simulink model "Levitador_aire_parametrizado"  (R2024b)
settings: Solver=VariableStepAuto  StartTime=0.0  StopTime=30  MaxStep=0.1  RelTol=1e-3
undefined symbols (not defined in the file): alfa, g, kd, kf, ki, kp, m, tao1, xi
libraries: slpidlib x1
settings Model: PacingRate=10  Creator=santiagolopez  LastModifiedBy=santiagolopez
settings DataIOCC: ReturnWorkspaceOutputs=off

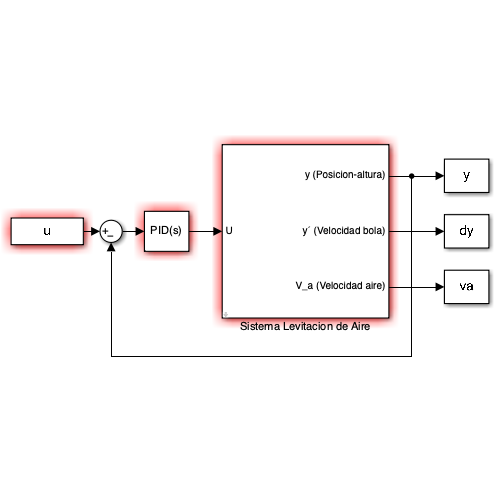
[thumbnail: Simulink's stored preview of the top-level diagram]
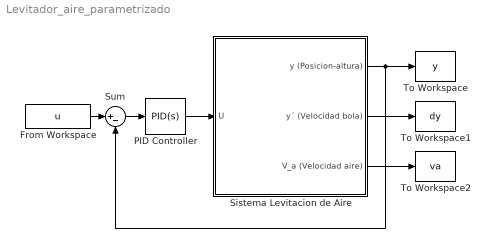
== system Levitador_aire_parametrizado ==
  From Workspace : FromWorkspace  VariableName=u
  PID Controller : slpidlib/PID Controller  Controller=PID  Form=Parallel  TimeDomain=Continuous-time  UseExternalTs=off  SampleTime=-1  IntegratorMethod=Forward Euler  FilterMethod=Forward Euler  ControllerParametersSource=internal  P=kp  I=ki  UseKiTs=off  D=kd  UseExternalDerivativeSource=off  N=100  UseFilter=on  TunerSelectOption=Transfer Function Based (PID Tuner App)  InitialConditionSource=internal  InitialConditionForIntegrator=0  InitialConditionForFilter=0  DifferentiatorICPrevScaledInput=0  ExternalReset=none  TrackingMode=off  Kt=1  LimitOutput=off  SatLimitsSource=internal  UpperSaturationLimit=inf  LowerSaturationLimit=-inf  LinearizeAsGain=on  AntiWindupMode=none  Kb=1  LimitIntegrator=off  UpperIntegratorSaturationLimit=inf  LowerIntegratorSaturationLimit=-inf  POutMin=[]  POutMax=[]  IOutMin=[]  IOutMax=[]  DOutMin=[]  DOutMax=[]  NOutMin=[]  NOutMax=[]  SumOutMin=[]  SumOutMax=[]  SaturationOutMin=[]  SaturationOutMax=[]  PParamMin=[]  PParamMax=[]  IParamMin=[]  IParamMax=[]  DParamMin=[]  DParamMax=[]  NParamMin=[]  NParamMax=[]  KbParamMin=[]  KbParamMax=[]  KtParamMin=[]  KtParamMax=[]  KbOutMin=[]  KbOutMax=[]  KtOutMin=[]  KtOutMax=[]  IntegratorOutMin=[]  IntegratorOutMax=[]  FilterOutMin=[]  FilterOutMax=[]  SumI1OutMin=[]  SumI1OutMax=[]  SumI2OutMin=[]  SumI2OutMax=[]  SumI3OutMin=[]  SumI3OutMax=[]  SumI4OutMin=[]  SumI4OutMax=[]  SumDOutMin=[]  SumDOutMax=[]  DifferentiatorOutMin=[]  DifferentiatorOutMax=[]  FilterDiffOutCoefMin=[]  FilterDiffOutCoefMax=[]  ReciprocalOutMin=[]  ReciprocalOutMax=[]  SumDenOutMin=[]  SumDenOutMax=[]  SumNumOutMin=[]  SumNumOutMax=[]  DivideOutMin=[]  DivideOutMax=[]  UdiffTsProdOutMin=[]  UdiffTsProdOutMax=[]  NTsProdOutMin=[]  NTsProdOutMax=[]  UintegralTsProdOutMin=[]  UintegralTsProdOutMax=[]  UngainTsProdOutMin=[]  UngainTsProdOutMax=[]  ClampingZeroOutDataTypeStr=Inherit: Inherit via back propagation  ClampingZeroOutMin=[]  ClampingZeroOutMax=[]  FilterDenConstantOutDataTypeStr=Inherit: Inherit via back propagation  FilterDenConstantOutMin=[]  FilterDenConstantOutMax=[]  PCopyOutDataTypeStr=Inherit: Inherit via back propagation  PCopyOutMin=[]  PCopyOutMax=[]  NCopyOutDataTypeStr=Inherit: Inherit via back propagation  NCopyOutMin=[]  NCopyOutMax=[]  IntegratorContinuousStateAttributes=''  IntegratorStateMustResolveToSignalObject=off  IntegratorRTWStateStorageClass=Auto  FilterContinuousStateAttributes=''  FilterStateMustResolveToSignalObject=off  FilterRTWStateStorageClass=Auto  ParallelPVariant=InternalParameters  IdealPVariant=Disabled  IVariant=InternalParameters  DVariant=InternalParameters  IntegratorVariant=Continuous  SatVariant=Disabled  AWVariant=Passthrough  PCopyVariant=Disabled  TRVariant=Disabled  FdbkBlocksVariant=Forward  IdealPFdbkVariant=Disabled  SatFdbkVariant=Disabled  DerivativeFilterVariant=ContFilter  NVariant=InternalParameters  NCopyVariant=Disabled  FilterICVariant=InternalICsFilter  IntegratorICVariant=InternalICs  ExternalResetVariant=Disabled  TRSumVariant=Passthrough  SumFdbkVariant=Disabled  SumVariant=Sum_PID  TsampFilterVariant=InternalTs  TsampNgainVariant=Passthrough  TsampIntegralVariant=Disabled_SignalSpec  ExternalSaturationOutDataTypeStr=Inherit: Same as second input  DerivativeSourceVariant=ErrorSignal  PreIntVariant=InternalPreInt
  Sistema Levitacion de Aire : Subsystem  mask{g=g, m=m, tao1=tao1, Kf=kf, alfa=alfa, ci=xi}
      mask prompts: g "Aceleracion de la gravedad (g, m/s^2)"; m "Masa (m, kg)"; tao1 "Constante de tiempo (tao1, s)"; Kf "Ganancia (Kf, m/s por unidad de entrada)"; alfa "Coeficiente aerodinamico (alfa,"; ci "Condiciones iniciales [y, y', v_a]"
  Sum : Sum  Inputs=|+-
  To Workspace : ToWorkspace  VariableName=y  SaveFormat=Timeseries  SampleTime=-1
  To Workspace1 : ToWorkspace  VariableName=dy  SaveFormat=Timeseries  SampleTime=-1
  To Workspace2 : ToWorkspace  VariableName=va  SaveFormat=Structure With Time  SampleTime=-1
  wires:
  Sistema Levitacion de Aire/1(y (Posicion-altura)) -> Sum/2, To Workspace/1
  Sistema Levitacion de Aire/2(y´ (Velocidad bola)) -> To Workspace1/1
  Sistema Levitacion de Aire/3(V_a (Velocidad aire)) -> To Workspace2/1
  From Workspace/1 -> Sum/1
  Sum/1 -> PID Controller/1
  PID Controller/1 -> Sistema Levitacion de Aire/1(U)

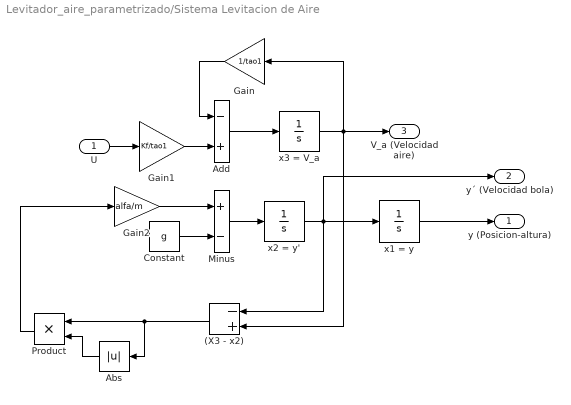
== system Levitador_aire_parametrizado/Sistema Levitacion de Aire ==
  U : Inport
  (X3 - x2) : Sum  Inputs=-+
  Abs : Abs  SaturateOnIntegerOverflow=off
  Add : Sum  Inputs=-+
  Constant : Constant  Value=g
  Gain : Gain  Gain=1/tao1
  Gain1 : Gain  Gain=Kf/tao1
  Gain2 : Gain  Gain=alfa/m
  Minus : Sum  Inputs=+-
  Product : Product
  x1 = y : Integrator  InitialCondition=ci(1)
  x2 = y' : Integrator  InitialCondition=ci(2)
  x3 = V_a : Integrator  InitialCondition=ci(3)
  y (Posicion-altura) : Outport
  y´ (Velocidad bola) : Outport  Port=2
  V_a (Velocidad aire) : Outport  Port=3
  wires:
  U/1 -> Gain1/1
  Constant/1 -> Minus/2
  Abs/1 -> Product/2
  Minus/1 -> x2 = y'/1
  Add/1 -> x3 = V_a/1
  Gain1/1 -> Add/2
  Gain/1 -> Add/1
  Gain2/1 -> Minus/1
  x2 = y'/1 -> y´ (Velocidad bola)/1, (X3 - x2)/1, x1 = y/1
  (X3 - x2)/1 -> Abs/1, Product/1
  x3 = V_a/1 -> Gain/1, V_a (Velocidad aire)/1, (X3 - x2)/2
  x1 = y/1 -> y (Posicion-altura)/1
  Product/1 -> Gain2/1
